simulink model "Double_current_Vin_Vout_integrator_method"  (R2024a)
settings: Solver=VariableStepAuto  StartTime=0.0  StopTime=10.0  RelTol=1e-3
values from neighbouring files (symbols this model uses):
  c1 = 20    [Double_current_parameters.mat]
  c2 = 50    [Double_current_parameters.mat]
  r1 = 200    [Double_current_parameters.mat]
  r2 = 1    [Double_current_parameters.mat]
settings Model: Creator=nassa  LastModifiedBy=nassa

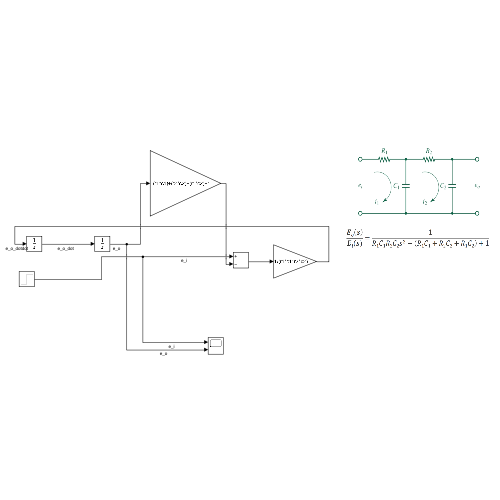
[thumbnail: Simulink's stored preview of the top-level diagram]
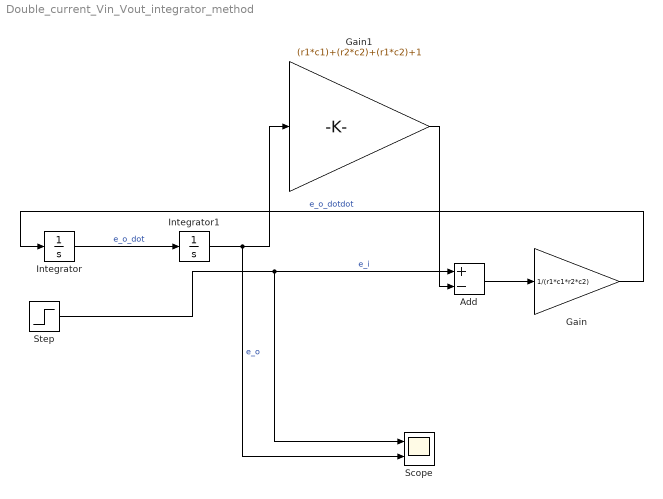
== system Double_current_Vin_Vout_integrator_method ==
  Add : Sum  Inputs=+-
  Gain : Gain  Gain=1/(r1*c1*r2*c2)
  Gain1 : Gain  Gain=(r1*c1)+(r2*c2)+(r1*c2)+1
  Integrator : Integrator
  Integrator1 : Integrator
  Scope : Scope  NumInputPorts=2
  Step : Step  SampleTime=0
  wires:
  Integrator/1 -> Integrator1/1  "e_o_dot"
  Gain/1 -> Integrator/1  "e_o_dotdot"
  Integrator1/1 -> Scope/2, Gain1/1  "e_o"
  Step/1 -> Scope/1, Add/1  "e_i"
  Gain1/1 -> Add/2
  Add/1 -> Gain/1
